simulink model "sim_playing"  (R2019b)
settings: Solver=ode4  StartTime=0.0  StopTime=10.0  FixedStep=0.01  RelTol=1e-3
values from neighbouring files (symbols this model uses):
  c = 1    [model_playing.m]
  k = 10    [model_playing.m]
  m = 1    [model_playing.m]
settings Model: Creator=Peanatsu  LastModifiedBy=Peanatsu

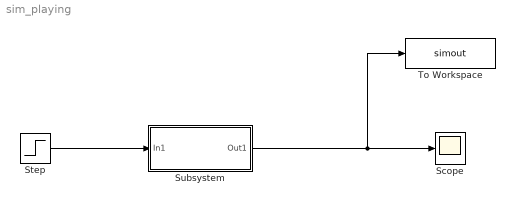
== system sim_playing ==
  Scope : Scope
  Step : Step  SampleTime=0
  Subsystem : Subsystem
  To Workspace : ToWorkspace  VariableName=simout  SaveFormat=Timeseries  SampleTime=-1
  wires:
  Step/1 -> Subsystem/1(In1)
  Subsystem/1(Out1) -> To Workspace/1, Scope/1

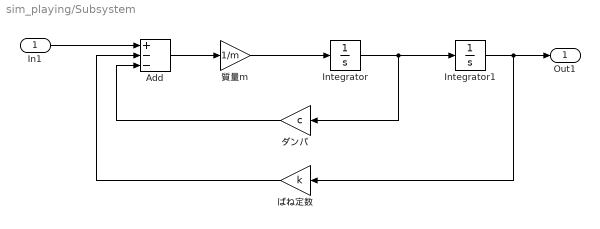
== system sim_playing/Subsystem ==
  In1 : Inport
  Add : Sum  Inputs=+--
  Integrator : Integrator
  Integrator1 : Integrator
  "ばね定数 " : Gain  Gain=k
  ダンパ : Gain  Gain=c
  質量m : Gain  Gain=1/m
  Out1 : Outport
  wires:
  Integrator/1 -> ダンパ/1, Integrator1/1
  Add/1 -> 質量m/1
  "ばね定数 "/1 -> Add/2
  ダンパ/1 -> Add/3
  In1/1 -> Add/1
  質量m/1 -> Integrator/1
  Integrator1/1 -> "ばね定数 "/1, Out1/1
